simulink model "hw03"  (R2021a)
settings: Solver=FixedStepAuto  StartTime=0.0  StopTime=14.4  FixedStep=1e-3  RelTol=1e-3
libraries: simulink x1
settings Model: Creator=Wasif  LastModifiedBy=Wasif

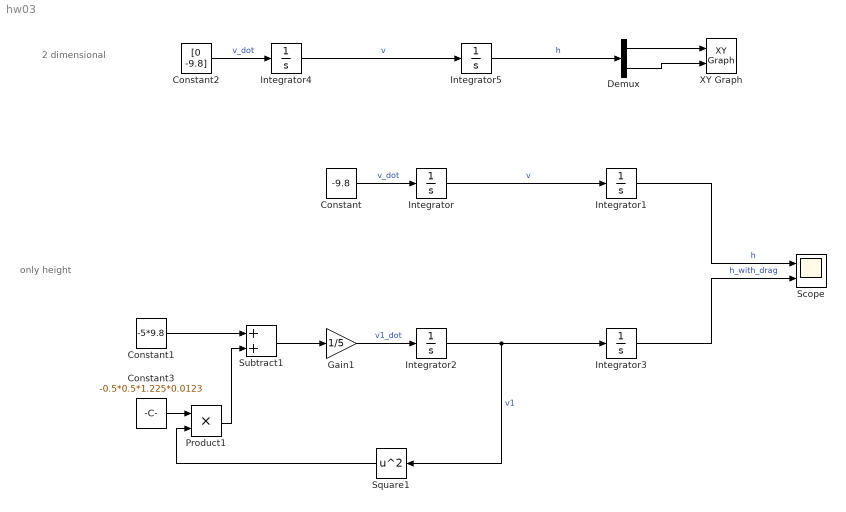
== system hw03 ==
  note: only height
  note: 2 dimensional
  Constant : Constant  Value=-9.8
  Constant1 : Constant  Value=-5*9.8
  Constant2 : Constant  Value=[0 -9.8]
  Constant3 : Constant  Value=-0.5*0.5*1.225*0.0123
  Demux : Demux  Outputs=2
  Gain1 : Gain  Gain=1/5
  Integrator : Integrator  InitialCondition=100*sind(45)
  Integrator1 : Integrator
  Integrator2 : Integrator  InitialCondition=100*sind(45)
  Integrator3 : Integrator
  Integrator4 : Integrator  InitialCondition=[100*cosd(45) 100*sind(45)]
  Integrator5 : Integrator  InitialCondition=[0 0]
  Product1 : Product
  Scope : Scope  NumInputPorts=2
  Square1 : Math  Operator=square  SaturateOnIntegerOverflow=on
  Subtract1 : Sum
  XY Graph : simulink/Sinks/XY Graph  xmin=0  xmax=1200  ymin=0  ymax=400  st=-1
  wires:
  Integrator/1 -> Integrator1/1  "v"
  Integrator1/1 -> Scope/1  "h"
  Constant/1 -> Integrator/1  "v_dot"
  Product1/1 -> Subtract1/2
  Integrator3/1 -> Scope/2  "h_with_drag"
  Subtract1/1 -> Gain1/1
  Gain1/1 -> Integrator2/1  "v1_dot"
  Square1/1 -> Product1/2
  Constant3/1 -> Product1/1
  Constant1/1 -> Subtract1/1
  Integrator2/1 -> Square1/1, Integrator3/1  "v1"
  Constant2/1 -> Integrator4/1  "v_dot"
  Integrator4/1 -> Integrator5/1  "v"
  Integrator5/1 -> Demux/1  "h"
  Demux/1 -> XY Graph/1
  Demux/2 -> XY Graph/2
